simulink model "gm_transmitter"  (R2020b)
settings: Solver=FixedStepDiscrete  StartTime=0.0  StopTime=100000  RelTol=1e-3
undefined symbols (not defined in the file or in its folder): message
libraries: hdlmdlgenlib x98, dspsigops x53, hdlsllib x22, simulink x11, dspmlti4 x2, whdlio x1
(part 1 of 3)
settings Model: Creator=wardo  LastModifiedBy=EFlores
settings DataIOCC: LimitDataPoints=on  SaveOutput=off  SaveTime=off
settings OptimizationCC: BlockReduction=off  ConditionallyExecuteInputs=off  DefaultParameterBehavior=Inlined  LifeSpan=inf
settings DebuggingCC: AlgebraicLoopMsg=error  InheritedTsInSrcMsg=none  SingleTaskRateTransMsg=error  AllowSymbolicDim=off  StrictBusMsg=ErrorOnBusTreatedAsVector  SFUnexpectedBacktrackingDiag=warning  SFNoUnconditionalDefaultTransitionDiag=warning  SFExecutionAtInitializationDiag=none  ArithmeticOperatorsInVariantConditions=warning
settings HardwareCC: ProdBitPerPointer=32  ProdBitPerSizeT=32  ProdBitPerPtrDiffT=32  ProdLargestAtomicFloat=None  ProdIntDivRoundTo=Undefined  ProdEndianess=Unspecified  ProdWordSize=32  ProdHWDeviceType=ASIC/FPGA->ASIC/FPGA  ProdEqTarget=off
settings SFSimCC: SimUseLocalCustomCode=off  CustomCodeUndefinedFunction=UseInterfaceOnly
settings RTWCC: RTWUseLocalCustomCode=off
settings CodeAppCC: StateflowObjectComments=on
settings GRTTargetCC: TargetLangStandard=C89/C90 (ANSI)
settings ConfigComp: CovScope=ReferencedModels  CovMetricSettings=dw  CovSaveCumulativeToWorkspaceVar=on  CovSaveSingleToWorkspaceVar=on  CovExternalEMLEnable=off  CovSFcnEnable=off

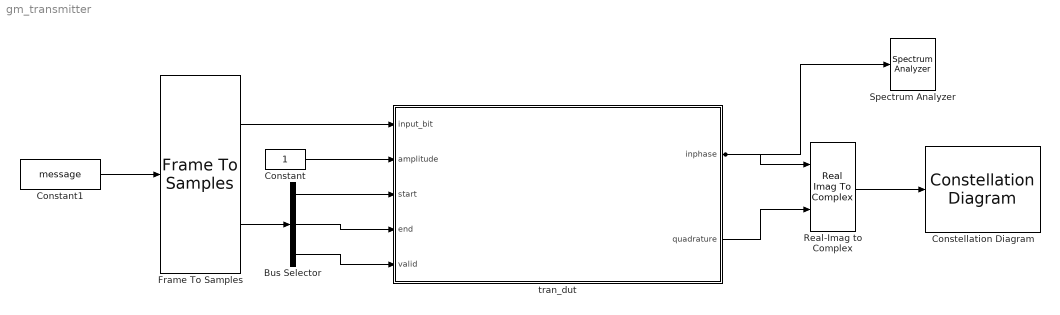
== system gm_transmitter ==
  Bus Selector : BusSelector  OutputSignals=start,end,valid
  Constant : Constant  OutDataTypeStr=uint8  SampleTime=-1
  Constant1 : Constant  Value=message  OutDataTypeStr=fixdt(0,1,0)  SampleTime=100000
  Constellation Diagram : ConstellationDiagram
  Frame To Samples : whdlio/Frame To Samples  InterSampleIdleCycles=0  InterFrameIdleCycles=0  OutputSize=1  InterleaveSamples=off
      settings: SourceProductBaseCode=LH
  Real-Imag to Complex : RealImagToComplex
  Spectrum Analyzer : SpectrumAnalyzer
  tran_dut : Subsystem
  wires:
  Bus Selector/3 -> tran_dut/5(valid)
  Bus Selector/2 -> tran_dut/4(end)
  Bus Selector/1 -> tran_dut/3(start)
  Frame To Samples/2 -> Bus Selector/1
  tran_dut/2(quadrature) -> Real-Imag to Complex/2
  tran_dut/1(inphase) -> Spectrum Analyzer/1, Real-Imag to Complex/1
  Real-Imag to Complex/1 -> Constellation Diagram/1
  Constant1/1 -> Frame To Samples/1
  Constant/1 -> tran_dut/2(amplitude)
  Frame To Samples/1 -> tran_dut/1(input_bit)

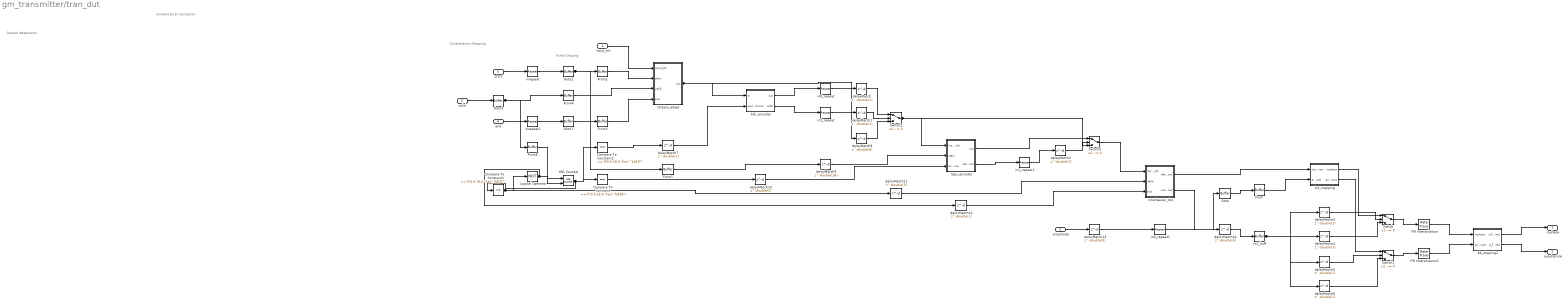
== system gm_transmitter/tran_dut ==
  note: Stream Adaptation
  note: Forward Error Correction
  note: Constellation Mapping
  note: Pulse Shaping
  input_bit : Inport  OutDataTypeStr=fixdt(0, 1, 0)  PortDimensions=1  SampleTime=2.06577425218972
  amplitude : Inport  Port=2  OutDataTypeStr=uint8  PortDimensions=1  SampleTime=2.06577425218972
  start : Inport  Port=3  OutDataTypeStr=boolean  PortDimensions=1  SampleTime=2.06577425218972
  end : Inport  Port=4  OutDataTypeStr=boolean  PortDimensions=1  SampleTime=2.06577425218972
  valid : Inport  Port=5  OutDataTypeStr=boolean  PortDimensions=1  SampleTime=2.06577425218972
  Compare To Constant : simulink/Logic and Bit Operations/Compare To Constant  relop===  const="fi(0,0,16,0,\"hex\",\"bdd8\")"  OutDataTypeStr=boolean
  Compare To Constant1 : simulink/Logic and Bit Operations/Compare To Constant  relop=<=  const="fi(0,0,16,0,\"hex\",\"fd20\")"  OutDataTypeStr=boolean
  Compare To Constant2 : simulink/Logic and Bit Operations/Compare To Constant  relop===  const="fi(0,0,16,0,\"hex\",\"bd18\")"  OutDataTypeStr=boolean
  FIR Interpolation : RateTransition  OutPortSampleTimeOpt=Multiple of input port sample time  OutPortSampleTimeMultiple=8
  FIR Interpolation1 : RateTransition  OutPortSampleTimeOpt=Multiple of input port sample time  OutPortSampleTimeMultiple=8
  From{,1..4,8} (6 alike) : hdlmdlgenlib/Buffer
      settings: SourceProductBaseCode=SL
  Goto{,1..3} (4 alike) : hdlmdlgenlib/Buffer
      settings: SourceProductBaseCode=SL
  HDL Counter : hdlsllib/Sources/HDL Counter  CountType=Count limited  CountInit=double(0)  CountStep=double(1)  CountMax=double(64800)  CountFromType=Initial value  CountFrom=double(0)  CountResetPort=on  CountLoadPort=off  CountEnbPort=on  CountDirPort=off  CountDataType=Unsigned  CountWordLen=16  CountFracLen=0  CountSampTime=2.06577425218972
  Logical Operator : Logic  Operator=NOT  Inputs=1  AllPortsSameDT=off  OutDataTypeStr=boolean  SampleTime=2.06577425218972
  Switch : Switch  Criteria=u2 ~= 0  Threshold=double(0)  OutDataTypeStr=fixdt(1, 25, 15)  SampleTime=0.258221781523715
  Switch1 : Switch  Criteria=u2 ~= 0  Threshold=double(0)  OutDataTypeStr=fixdt(1, 25, 15)  SampleTime=0.258221781523715
  Switch2 : Switch  Criteria=u2 ~= 0  Threshold=double(0)  OutDataTypeStr=boolean  SampleTime=0.258221781523715
  Switch3 : Switch  Criteria=u2 ~= 0  Threshold=double(0)  OutDataTypeStr=boolean  SampleTime=0.258221781523715
  bb_shaping1 : Subsystem
  bch_encoder : Subsystem
  bit_mapping : Subsystem
  delayMatch{,1..6} (7 alike) : Delay  DelayLength=double(1)  InitialCondition=0  SampleTime=0.258221781523715
  delayMatch10 : Delay  DelayLength=double(2)  InitialCondition=0  SampleTime=2.06577425218972
  delayMatch11 : Delay  DelayLength=double(2)  InitialCondition=0  SampleTime=2.06577425218972
  delayMatch12 : Delay  DelayLength=double(2)  InitialCondition=0  SampleTime=2.06577425218972
  delayMatch13 : Delay  DelayLength=double(3)  InitialCondition=0  SampleTime=2.06577425218972
  delayMatch14 : Delay  DelayLength=double(8)  InitialCondition=0  SampleTime=0.258221781523715
  delayMatch7 : Delay  DelayLength=double(1)  InitialCondition=0  SampleTime=2.06577425218972
  delayMatch8 : Delay  DelayLength=double(8)  InitialCondition=0  SampleTime=0.258221781523715
  delayMatch9 : Delay  DelayLength=double(16)  InitialCondition=0  SampleTime=0.258221781523715
  in0_repeat : dspsigops/Repeat  N=double(8)  RateOptions=Allow multirate processing  ic=0  mode=Unused parameter value
  in0_repeat1 : dspsigops/Repeat  N=double(8)  RateOptions=Allow multirate processing  ic=0  mode=Unused parameter value
  in1_repeat : dspsigops/Repeat  N=double(8)  RateOptions=Allow multirate processing  ic=0  mode=Unused parameter value
  in1_repeat1 : dspsigops/Repeat  N=double(8)  RateOptions=Allow multirate processing  ic=0  mode=Unused parameter value
  in2_buff : hdlmdlgenlib/Buffer
      settings: SourceProductBaseCode=SL
  inrepeat : dspsigops/Repeat  N=double(8)  RateOptions=Allow multirate processing  ic=0  mode=Unused parameter value
  inrepeat1 : dspsigops/Repeat  N=double(8)  RateOptions=Allow multirate processing  ic=0  mode=Unused parameter value
  interleaver_dut : Subsystem
  ldpc_encoder : Subsystem
  stream_adapt : Subsystem
  inphase : Outport  VectorParamsAs1DForOutWhenUnconnected=off
  quadrature : Outport  Port=2  VectorParamsAs1DForOutWhenUnconnected=off
  wires:
  input_bit/1 -> stream_adapt/1(input_bit)
  delayMatch13/1 -> in0_repeat1/1
  start/1 -> inrepeat/1
  end/1 -> inrepeat1/1
  valid/1 -> Goto3/1
  HDL Counter/1 -> Compare To Constant1/1, Compare To Constant2/1, Compare To Constant/1
  bb_shaping1/1(i_filtered) -> inphase/1
  bb_shaping1/2(q_filtered) -> quadrature/1
  bch_encoder/1(out) -> in0_repeat/1
  bch_encoder/2(valid) -> in1_repeat/1
  interleaver_dut/1(data_out) -> bit_mapping/1(input_sequence)
  delayMatch14/1 -> in2_buff/1
  ldpc_encoder/1(out) -> Switch3/1
  ldpc_encoder/2(valid_out) -> in1_repeat1/1
  delayMatch8/1 -> Switch2/3
  From2/1 -> stream_adapt/2(start)
  delayMatch9/1 -> ldpc_encoder/2(start)
  From4/1 -> stream_adapt/3(valid)
  From8/1 -> HDL Counter/2
  From3/1 -> stream_adapt/4(end)
  delayMatch11/1 -> interleaver_dut/2(valid)
  delayMatch12/1 -> interleaver_dut/3(end)
  delayMatch7/1 -> bch_encoder/2(end_of_frame)
  Switch2/1 -> ldpc_encoder/1(input_bit), Switch3/3
  delayMatch10/1 -> ldpc_encoder/3(end_of_frame)
  Switch3/1 -> interleaver_dut/1(input_bit)
  FIR Interpolation/1 -> bb_shaping1/1(inphase)
  FIR Interpolation1/1 -> bb_shaping1/2(quadrature)
  Compare To Constant2/1 -> delayMatch7/1
  stream_adapt/1(out) -> delayMatch8/1, bch_encoder/1(in)
  From1/1 -> delayMatch9/1
  Compare To Constant/1 -> delayMatch10/1
  Compare To Constant1/1 -> delayMatch11/1, Logical Operator/1
  Logical Operator/1 -> delayMatch12/1, HDL Counter/1
  amplitude/1 -> delayMatch13/1
  interleaver_dut/2(valid_out) -> delayMatch14/1
  inrepeat/1 -> Goto2/1
  Goto2/1 -> From2/1, From1/1
  Goto3/1 -> From8/1, From4/1
  inrepeat1/1 -> Goto1/1
  Goto1/1 -> From3/1
  in0_repeat/1 -> delayMatch/1
  in1_repeat/1 -> delayMatch1/1
  delayMatch/1 -> Switch2/1
  delayMatch1/1 -> Switch2/2
  in1_repeat1/1 -> delayMatch2/1
  delayMatch2/1 -> Switch3/2
  Switch/1 -> FIR Interpolation/1
  Switch1/1 -> FIR Interpolation1/1
  in0_repeat1/1 -> Goto/1
  Goto/1 -> From/1
  From/1 -> bit_mapping/2(amplitude)
  bit_mapping/1(inphase) -> Switch/1
  bit_mapping/2(quadrature) -> Switch1/1
  delayMatch3/1 -> Switch/2
  delayMatch4/1 -> Switch/3
  delayMatch5/1 -> Switch1/2
  delayMatch6/1 -> Switch1/3
  in2_buff/1 -> delayMatch6/1, delayMatch5/1, delayMatch4/1, delayMatch3/1

== system gm_transmitter/tran_dut/bb_shaping1 ==
  inphase : Inport  OutDataTypeStr=fixdt(1, 25, 15)  PortDimensions=1  SampleTime=2.06577425218972
  quadrature : Inport  Port=2  OutDataTypeStr=fixdt(1, 25, 15)  PortDimensions=1  SampleTime=2.06577425218972
  FIR Interpolation : dspmlti4/FIR Interpolation  FilterSource=Dialog parameters  PrivateCoeffs=0  h=[-0.00599670410156250,-0.00514221191406250,-0.00289916992187500,0.000442504882812500,0.00431823730468750,0.00794982910156250,0.0104980468750000,0.0112304687500000,0.00967407226562500,0.00578308105468750,0,-0.00680541992187500,-0.0134124755859375,-0.0184326171875000,-0.0205841064453125,-0.0189819335937500,-0.0133361816406250,-0.00410461425781250,0.00752258300781250,0.0196380615234375,0.0300140380859375,0.0363464355468750,0.0367584228515625,0.0301208496093750,0.0164794921875000,-0.00291442871093750,-0.0254821777343750,-0.0476837158203125,-0.0653228759765625,-0.0742187500000000,-0.0707244873046875,-0.0524291992187500,-0.0185852050781250,0.0296783447265625,0.0892028808593750,0.155227661132813,0.221755981445313,0.282333374023438,0.330810546875000,0.362121582031250,0.372940063476563,0.362121582031250,0.330810546875000,0.282333374023438,0.221755981445313,0.155227661132813,0.0892028808593750,0.0296783447265625,-0.0185852050781250,-0.0524291992187500,-0.0707244873046875,-0.0742187500000000,-0.0653228759765625,-0.0476837158203125,-0.0254821777343750,-0.00291442871093750,0.0164794921875000,0.0301208496093750,0.0367584228515625,0.0363464355468750,0.0300140380859375,0.0196380615234375,0.00752258300781250,-0.00410461425781250,-0.0133361816406250,-0.0189819335937500,-0.0205841064453125,-0.0184326171875000,-0.0134124755859375,-0.00680541992187500,0,0.00578308105468750,0.00967407226562500,0.0112304687500000,0.0104980468750000,0.00794982910156250,0.00431823730468750,0.000442504882812500,-0.00289916992187500,-0.00514221191406250,-0.00599670410156250]  L=8  FilterObject=FINTERP  framing=Allow multirate processing  outputBufInitCond=0  roundingMode=Floor  overflowMode=off  firstCoeffMode=Specify word length  firstCoeffWordLength=16  firstCoeffFracLength=15  firstCoeffDataTypeStr=fixdt(1,16)  firstCoeffMin=[]  firstCoeffMax=[]  firstCoeffLastDataTypeStr=fixdt(1,16)  outputDataTypeStr=Inherit: Same as accumulator  outputMin=[]  outputMax=[]  outputLastDataTypeStr=Inherit: Same as accumulator
      settings: SourceProductName=DSP System Toolbox
  FIR Interpolation1 : dspmlti4/FIR Interpolation  FilterSource=Dialog parameters  PrivateCoeffs=0  h=[-0.00599670410156250,-0.00514221191406250,-0.00289916992187500,0.000442504882812500,0.00431823730468750,0.00794982910156250,0.0104980468750000,0.0112304687500000,0.00967407226562500,0.00578308105468750,0,-0.00680541992187500,-0.0134124755859375,-0.0184326171875000,-0.0205841064453125,-0.0189819335937500,-0.0133361816406250,-0.00410461425781250,0.00752258300781250,0.0196380615234375,0.0300140380859375,0.0363464355468750,0.0367584228515625,0.0301208496093750,0.0164794921875000,-0.00291442871093750,-0.0254821777343750,-0.0476837158203125,-0.0653228759765625,-0.0742187500000000,-0.0707244873046875,-0.0524291992187500,-0.0185852050781250,0.0296783447265625,0.0892028808593750,0.155227661132813,0.221755981445313,0.282333374023438,0.330810546875000,0.362121582031250,0.372940063476563,0.362121582031250,0.330810546875000,0.282333374023438,0.221755981445313,0.155227661132813,0.0892028808593750,0.0296783447265625,-0.0185852050781250,-0.0524291992187500,-0.0707244873046875,-0.0742187500000000,-0.0653228759765625,-0.0476837158203125,-0.0254821777343750,-0.00291442871093750,0.0164794921875000,0.0301208496093750,0.0367584228515625,0.0363464355468750,0.0300140380859375,0.0196380615234375,0.00752258300781250,-0.00410461425781250,-0.0133361816406250,-0.0189819335937500,-0.0205841064453125,-0.0184326171875000,-0.0134124755859375,-0.00680541992187500,0,0.00578308105468750,0.00967407226562500,0.0112304687500000,0.0104980468750000,0.00794982910156250,0.00431823730468750,0.000442504882812500,-0.00289916992187500,-0.00514221191406250,-0.00599670410156250]  L=8  FilterObject=FINTERP  framing=Allow multirate processing  outputBufInitCond=0  roundingMode=Floor  overflowMode=off  firstCoeffMode=Specify word length  firstCoeffWordLength=16  firstCoeffFracLength=15  firstCoeffDataTypeStr=fixdt(1,16)  firstCoeffMin=[]  firstCoeffMax=[]  firstCoeffLastDataTypeStr=fixdt(1,16)  outputDataTypeStr=Inherit: Same as accumulator  outputMin=[]  outputMax=[]  outputLastDataTypeStr=Inherit: Same as accumulator
      settings: SourceProductName=DSP System Toolbox
  i_filtered : Outport  VectorParamsAs1DForOutWhenUnconnected=off
  q_filtered : Outport  Port=2  VectorParamsAs1DForOutWhenUnconnected=off
  wires:
  FIR Interpolation/1 -> i_filtered/1
  FIR Interpolation1/1 -> q_filtered/1
  inphase/1 -> FIR Interpolation/1
  quadrature/1 -> FIR Interpolation1/1

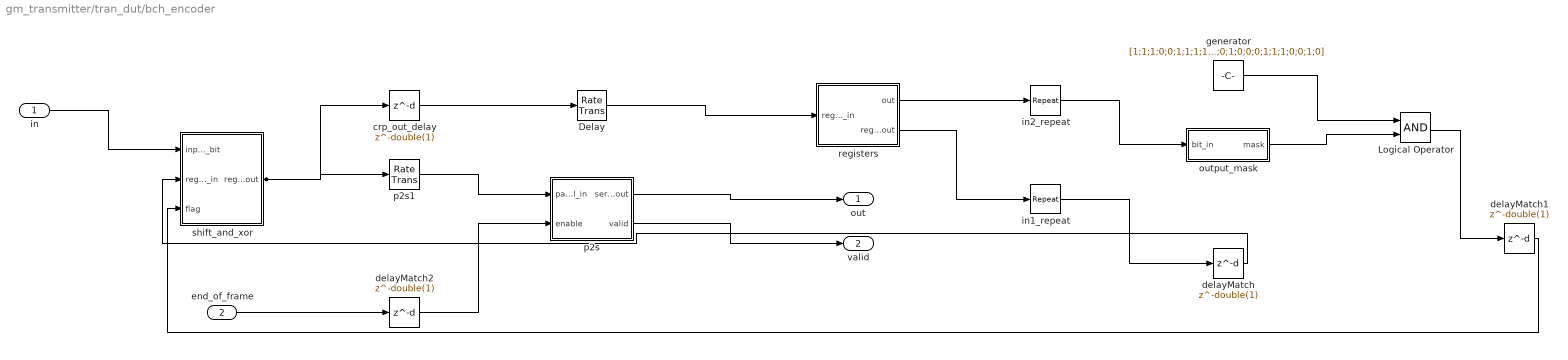
== system gm_transmitter/tran_dut/bch_encoder ==
  in : Inport  OutDataTypeStr=boolean  PortDimensions=1  SampleTime=0.258221781523715
  end_of_frame : Inport  Port=2  OutDataTypeStr=boolean  PortDimensions=1  SampleTime=2.06577425218972
  Delay : RateTransition  OutPortSampleTimeOpt=Multiple of input port sample time  OutPortSampleTimeMultiple=8
  Logical Operator : Logic  AllPortsSameDT=off  OutDataTypeStr=fixdt(0, 1, 0)  SampleTime=0.258221781523715
  crp_out_delay : Delay  DelayLength=double(1)  InitialCondition=0  SampleTime=0.258221781523715
  delayMatch : Delay  DelayLength=double(1)  InitialCondition=0  SampleTime=0.258221781523715
  delayMatch1 : Delay  DelayLength=double(1)  InitialCondition=0  SampleTime=0.258221781523715
  delayMatch2 : Delay  DelayLength=double(1)  InitialCondition=0  SampleTime=2.06577425218972
  generator : Constant  Value=[1;1;1;0;0;1;1;1;1;0;1;0;1;0;1;0;0;1;0;0;0;0;0;0;0;1;1;0;0;1;1;0;1;1;1;0;1;1;1;1;1;0;1;0;0;0;0;1;1;1;1;0;0;0;1;0;1;1;0;0;0;0;0;0;1;0;0;1;0;0;0;1;0;0;0;1;0;0;0;0;1;0;1;0;1;1;0;0;0;0;1;1;1;0;1;1;0;0;0;1;1;0;1;1;0;0;1;1;0;1;0;0;1;1;1;1;0;0;1;1;0;0;0;0;1;0;1;0;0;0;1;1;1;0;0;0;1;0;0;0;1;0;1;0;0;0;1;1;1;0;1;0;0;0;1;0;0;0;0;1;1;1;0;0;0;0;0;1;0;1;1;1;0;0;0;0;0;1;1;0;0;1;0;0;0;1;1;1;0;0;1;0]  OutDataTypeStr=fixdt(0, 1, 0)  SampleTime=0.258221781523715
  in1_repeat : dspsigops/Repeat  N=double(8)  RateOptions=Allow multirate processing  ic=0  mode=Unused parameter value
  in2_repeat : dspsigops/Repeat  N=double(8)  RateOptions=Allow multirate processing  ic=0  mode=Unused parameter value
  output_mask : Subsystem
  p2s : Subsystem
  p2s1 : RateTransition  OutPortSampleTimeOpt=Multiple of input port sample time  OutPortSampleTimeMultiple=8
  registers : Subsystem
  shift_and_xor : Subsystem
  out : Outport  VectorParamsAs1DForOutWhenUnconnected=off
  valid : Outport  Port=2  VectorParamsAs1DForOutWhenUnconnected=off
  wires:
  p2s/1(serial_out) -> out/1
  p2s/2(valid) -> valid/1
  delayMatch2/1 -> p2s/2(enable)
  in/1 -> shift_and_xor/1(input_bit)
  end_of_frame/1 -> delayMatch2/1
  registers/1(out) -> in2_repeat/1
  registers/2(registers_out) -> in1_repeat/1
  Delay/1 -> registers/1(registers_in)
  p2s1/1 -> p2s/1(parallel_in)
  crp_out_delay/1 -> Delay/1
  shift_and_xor/1(registers_out) -> p2s1/1, crp_out_delay/1
  in1_repeat/1 -> delayMatch/1
  in2_repeat/1 -> output_mask/1(bit_in)
  generator/1 -> Logical Operator/1
  output_mask/1(mask) -> Logical Operator/2
  delayMatch1/1 -> shift_and_xor/3(flag)
  delayMatch/1 -> shift_and_xor/2(registers_in)
  Logical Operator/1 -> delayMatch1/1

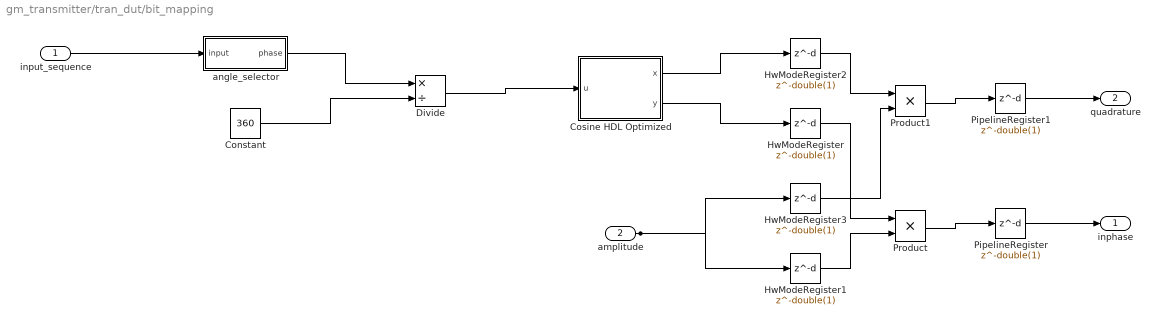
== system gm_transmitter/tran_dut/bit_mapping ==
  input_sequence : Inport  OutDataTypeStr=fixdt(0, 3, 0)  PortDimensions=1  SampleTime=0.258221781523715
  amplitude : Inport  Port=2  OutDataTypeStr=uint8  PortDimensions=1  SampleTime=0.258221781523715
  Constant : Constant  Value=360  OutDataTypeStr=fixdt(0, 9, 0)  SampleTime=0.258221781523715
  Cosine HDL Optimized : Subsystem  mask(Sine and Cosine HDL optimized block){OutputFormula=sin(2*pi*u) and cos(2*pi*u), NumDataPoints=double(32), TableDataTypeStr=fixdt(1,16,15), SimulateLUTROMDelay=off}
      mask prompts: OutputFormula "Simulink:masks:OutputFormula_MP"; NumDataPoints "HDLShared:hdlshared:CosineHDL_Npts"; TableDataTypeStr "Simulink:blkprm_prompts:TABLE_UNIFIEDDATATYPE"; SimulateLUTROMDelay "HDLShared:hdlshared:CosineHDL_Map2RAM"
      mask help: Sine and Cosine HDL optimized block using quarter wave symmetry, and HDL friendly settings.
      mask Help: helpview([docroot '/hdlcoder/helptargets.map'],'SineAndCosineHDL_Optimized');
      mask TypeOptions OutputFormula: sin(2*pi*u) | cos(2*pi*u) | exp(j*2*pi*u) | sin(2*pi*u) and cos(2*pi*u)
      mask Display:
      | port_label('input',1,'u')
      | port_label('output',1,'sin(2*pi*u)')
      | port_label('output',2,'cos(2*pi*u)')
      | xpos = 0.35;
      | yoffset = 0.5;
      | if ( SimulateLUTROMDelay )
      |   text(xpos,yoffset,'HDL (Z^{-1})','texmode','on')
      | else
      |    text(xpos,yoffset,'HDL')
      | end
  Divide : Product  Inputs=*/  OutDataTypeStr=fixdt(1, 16, 14)  RndMeth=Zero  SaturateOnIntegerOverflow=on  SampleTime=0.258221781523715
  HwModeRegister{,1..3} (4 alike) : Delay  DelayLength=double(1)  InitialCondition=0  SampleTime=0.258221781523715
  PipelineRegister : Delay  DelayLength=double(1)  InitialCondition=0  SampleTime=0.258221781523715
  PipelineRegister1 : Delay  DelayLength=double(1)  InitialCondition=0  SampleTime=0.258221781523715
  Product : Product  Inputs=**  OutDataTypeStr=fixdt(1, 25, 15)  SampleTime=0.258221781523715
  Product1 : Product  Inputs=**  OutDataTypeStr=fixdt(1, 25, 15)  SampleTime=0.258221781523715
  angle_selector : Subsystem
  inphase : Outport  VectorParamsAs1DForOutWhenUnconnected=off
  quadrature : Outport  Port=2  VectorParamsAs1DForOutWhenUnconnected=off
  wires:
  Constant/1 -> Divide/2
  Cosine HDL Optimized/1(x) -> HwModeRegister2/1
  Cosine HDL Optimized/2(y) -> HwModeRegister/1
  Divide/1 -> Cosine HDL Optimized/1(u)
  PipelineRegister/1 -> inphase/1
  PipelineRegister1/1 -> quadrature/1
  angle_selector/1(phase) -> Divide/1
  input_sequence/1 -> angle_selector/1(input)
  amplitude/1 -> HwModeRegister1/1, HwModeRegister3/1
  Product/1 -> PipelineRegister/1
  HwModeRegister/1 -> Product/1
  HwModeRegister1/1 -> Product/2
  Product1/1 -> PipelineRegister1/1
  HwModeRegister2/1 -> Product1/1
  HwModeRegister3/1 -> Product1/2

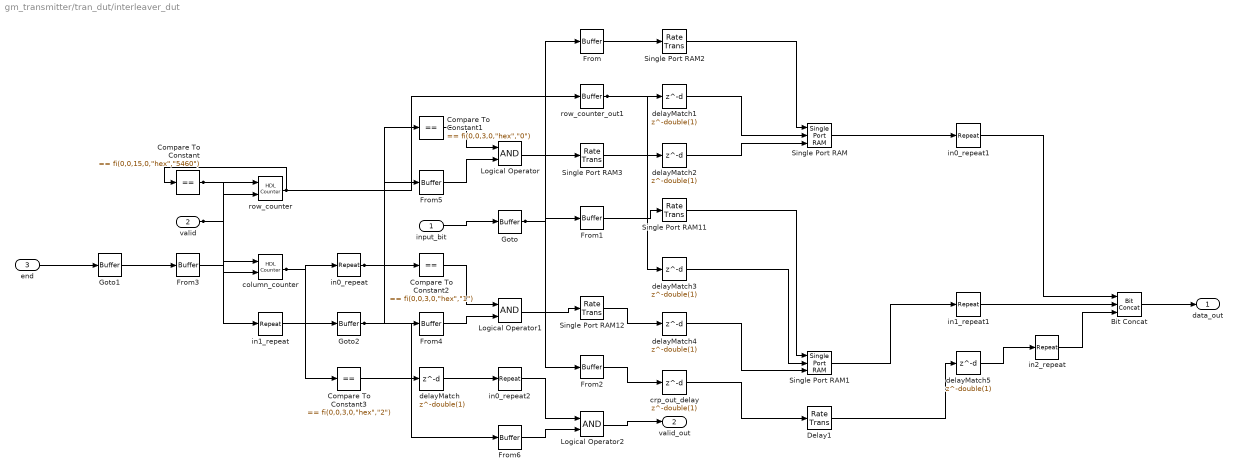
== system gm_transmitter/tran_dut/interleaver_dut ==
  input_bit : Inport  OutDataTypeStr=boolean  PortDimensions=1  SampleTime=0.258221781523715
  valid : Inport  Port=2  OutDataTypeStr=boolean  PortDimensions=1  SampleTime=2.06577425218972
  end : Inport  Port=3  OutDataTypeStr=boolean  PortDimensions=1  SampleTime=2.06577425218972
  Bit Concat : hdlsllib/Logic and Bit Operations/Bit Concat  numInputs=3
  Compare To Constant : simulink/Logic and Bit Operations/Compare To Constant  relop===  const="fi(0,0,15,0,\"hex\",\"5460\")"  OutDataTypeStr=boolean
  Compare To Constant1 : simulink/Logic and Bit Operations/Compare To Constant  relop===  const="fi(0,0,3,0,\"hex\",\"0\")"  OutDataTypeStr=boolean
  Compare To Constant2 : simulink/Logic and Bit Operations/Compare To Constant  relop===  const="fi(0,0,3,0,\"hex\",\"1\")"  OutDataTypeStr=boolean
  Compare To Constant3 : simulink/Logic and Bit Operations/Compare To Constant  relop===  const="fi(0,0,3,0,\"hex\",\"2\")"  OutDataTypeStr=boolean
  Delay1 : RateTransition  OutPortSampleTimeOpt=Multiple of input port sample time  OutPortSampleTimeMultiple=8
  From{,1..6} (7 alike) : hdlmdlgenlib/Buffer
      settings: SourceProductBaseCode=SL
  Goto : hdlmdlgenlib/Buffer
      settings: SourceProductBaseCode=SL
  Goto1 : hdlmdlgenlib/Buffer
      settings: SourceProductBaseCode=SL
  Goto2 : hdlmdlgenlib/Buffer
      settings: SourceProductBaseCode=SL
  Logical Operator : Logic  AllPortsSameDT=off  OutDataTypeStr=boolean  SampleTime=0.258221781523715
  Logical Operator1 : Logic  AllPortsSameDT=off  OutDataTypeStr=boolean  SampleTime=0.258221781523715
  Logical Operator2 : Logic  AllPortsSameDT=off  OutDataTypeStr=boolean  SampleTime=0.258221781523715
  Single Port RAM : hdlsllib/HDL RAMs/Single Port RAM  ram_size=15  dout_type=New data
      settings: SourceProductBaseCode=SL
  Single Port RAM1 : hdlsllib/HDL RAMs/Single Port RAM  ram_size=15  dout_type=New data
      settings: SourceProductBaseCode=SL
  Single Port RAM{2..3,11..12} (4 alike) : RateTransition  OutPortSampleTimeOpt=Multiple of input port sample time  OutPortSampleTimeMultiple=8
  column_counter : hdlsllib/Sources/HDL Counter  CountType=Count limited  CountInit=double(0)  CountStep=double(1)  CountMax=double(2)  CountFromType=Initial value  CountFrom=double(0)  CountResetPort=on  CountLoadPort=off  CountEnbPort=on  CountDirPort=off  CountDataType=Unsigned  CountWordLen=3  CountFracLen=0  CountSampTime=2.06577425218972
  crp_out_delay : Delay  DelayLength=double(1)  InitialCondition=0  SampleTime=0.258221781523715
  delayMatch{,1..5} (6 alike) : Delay  DelayLength=double(1)  InitialCondition=0  SampleTime=2.06577425218972
  in0_repeat : dspsigops/Repeat  N=double(8)  RateOptions=Allow multirate processing  ic=0  mode=Unused parameter value
  in0_repeat1 : dspsigops/Repeat  N=double(8)  RateOptions=Allow multirate processing  ic=0  mode=Unused parameter value
  in0_repeat2 : dspsigops/Repeat  N=double(8)  RateOptions=Allow multirate processing  ic=0  mode=Unused parameter value
  in1_repeat : dspsigops/Repeat  N=double(8)  RateOptions=Allow multirate processing  ic=0  mode=Unused parameter value
  in1_repeat1 : dspsigops/Repeat  N=double(8)  RateOptions=Allow multirate processing  ic=0  mode=Unused parameter value
  in2_repeat : dspsigops/Repeat  N=double(8)  RateOptions=Allow multirate processing  ic=0  mode=Unused parameter value
  row_counter : hdlsllib/Sources/HDL Counter  CountType=Count limited  CountInit=double(1)  CountStep=double(1)  CountMax=double(21600)  CountFromType=Initial value  CountFrom=double(1)  CountResetPort=on  CountLoadPort=off  CountEnbPort=on  CountDirPort=off  CountDataType=Unsigned  CountWordLen=15  CountFracLen=0  CountSampTime=2.06577425218972
  row_counter_out1 : hdlmdlgenlib/Buffer
      settings: SourceProductBaseCode=SL
  data_out : Outport  VectorParamsAs1DForOutWhenUnconnected=off
  valid_out : Outport  Port=2  VectorParamsAs1DForOutWhenUnconnected=off
  wires:
  delayMatch/1 -> in0_repeat2/1
  delayMatch5/1 -> in2_repeat/1
  Single Port RAM/1 -> in0_repeat1/1
  Single Port RAM1/1 -> in1_repeat1/1
  column_counter/1 -> in0_repeat/1, Compare To Constant3/1
  delayMatch1/1 -> Single Port RAM/2
  From3/1 -> column_counter/1
  delayMatch2/1 -> Single Port RAM/3
  delayMatch4/1 -> Single Port RAM1/3
  From6/1 -> Logical Operator2/2
  Bit Concat/1 -> data_out/1
  Logical Operator2/1 -> valid_out/1
  Single Port RAM2/1 -> Single Port RAM/1
  Single Port RAM11/1 -> Single Port RAM1/1
  input_bit/1 -> Goto/1
  valid/1 -> row_counter/2, in1_repeat/1
  end/1 -> Goto1/1
  delayMatch3/1 -> Single Port RAM1/2
  Single Port RAM3/1 -> delayMatch2/1
  row_counter_out1/1 -> delayMatch3/1, delayMatch1/1
  Single Port RAM12/1 -> delayMatch4/1
  Delay1/1 -> delayMatch5/1
  Compare To Constant/1 -> row_counter/1, column_counter/2
  row_counter/1 -> row_counter_out1/1, Compare To Constant/1
  From/1 -> Single Port RAM2/1
  From1/1 -> Single Port RAM11/1
  crp_out_delay/1 -> Delay1/1
  Goto/1 -> From2/1, From1/1, From/1
  From2/1 -> crp_out_delay/1
  Goto1/1 -> From3/1
  Logical Operator/1 -> Single Port RAM3/1
  Logical Operator1/1 -> Single Port RAM12/1
  in0_repeat/1 -> Compare To Constant2/1, Compare To Constant1/1
  in1_repeat/1 -> Goto2/1
  Compare To Constant1/1 -> Logical Operator/1
  Goto2/1 -> From6/1, From5/1, From4/1
  From5/1 -> Logical Operator/2
  Compare To Constant2/1 -> Logical Operator1/1
  From4/1 -> Logical Operator1/2
  in0_repeat1/1 -> Bit Concat/1
  in1_repeat1/1 -> Bit Concat/2
  in2_repeat/1 -> Bit Concat/3
  Compare To Constant3/1 -> delayMatch/1
  in0_repeat2/1 -> Logical Operator2/1

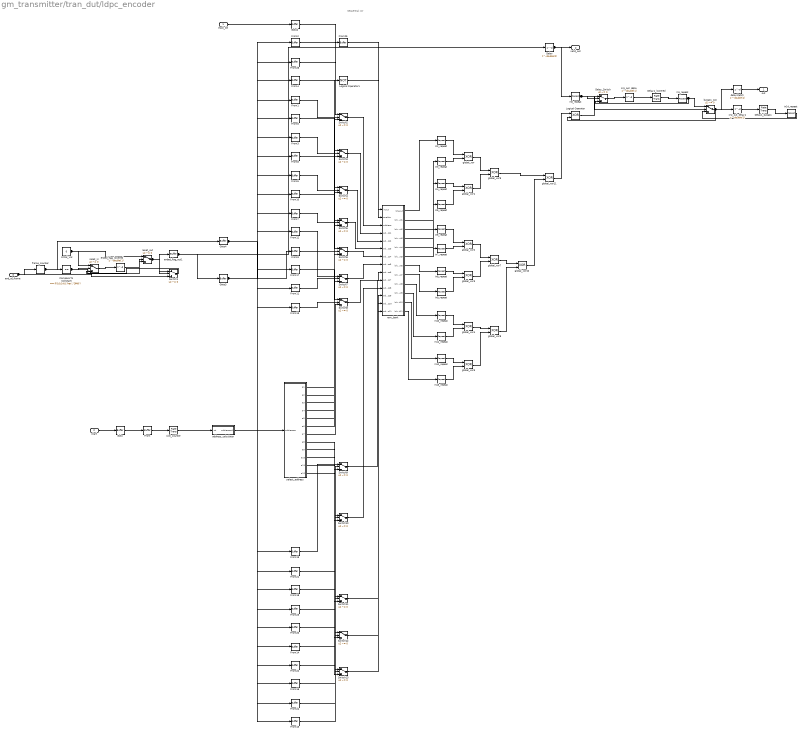
== system gm_transmitter/tran_dut/ldpc_encoder ==
  note: Sequential xor
  input_bit : Inport  OutDataTypeStr=boolean  PortDimensions=1  SampleTime=0.258221781523715
  start : Inport  Port=2  OutDataTypeStr=boolean  PortDimensions=1  SampleTime=0.258221781523715
  end_of_frame : Inport  Port=3  OutDataTypeStr=boolean  PortDimensions=1  SampleTime=2.06577425218972
  Compare To Constant : simulink/Logic and Bit Operations/Compare To Constant  relop===  const="fi(0,0,14,0,\"hex\",\"3f48\")"  OutDataTypeStr=boolean
  Delay : Delay  DelayLength=double(2)  InitialCondition=0  SampleTime=2.06577425218972
  Delay1_bypass : RateTransition  OutPortSampleTimeOpt=Multiple of input port sample time  OutPortSampleTimeMultiple=8
  Delay1_lowered : RateTransition  OutPortSampleTimeOpt=Multiple of input port sample time  OutPortSampleTimeMultiple=8
  Delay_Switch : Switch  Criteria=u2 ~= 0  Threshold=double(0)  OutDataTypeStr=fixdt(0, 1, 0)  SampleTime=0.258221781523715
  From{,1..26} (27 alike) : hdlmdlgenlib/Buffer
      settings: SourceProductBaseCode=SL
  Goto{,2..4} (4 alike) : hdlmdlgenlib/Buffer
      settings: SourceProductBaseCode=SL
  Initial_Val : Constant  Value=0  OutDataTypeStr=boolean  SampleTime=2.06577425218972
  Logical Operator : Logic  Operator=XOR  AllPortsSameDT=off  OutDataTypeStr=fixdt(0, 1, 0)  SampleTime=0.258221781523715
  Logical Operator1 : Logic  Operator=NOT  Inputs=1  AllPortsSameDT=off  OutDataTypeStr=boolean  SampleTime=2.06577425218972
  Switch1 : Switch  Criteria=u2 ~= 0  Threshold=double(0)  OutDataTypeStr=boolean  SampleTime=2.06577425218972
  Switch{2..13} (12 alike) : Switch  Criteria=u2 ~= 0  Threshold=double(0)  OutDataTypeStr=fixdt(0, 14, 0)  SampleTime=2.06577425218972
  address_calculator : Subsystem
  bypass_out : Switch  Criteria=u2 ~= 0  Threshold=double(0)  OutDataTypeStr=fixdt(0, 1, 0)  SampleTime=0.258221781523715
  crp_out_delay : Delay  DelayLength=double(1)  InitialCondition=0  SampleTime=0.258221781523715
  crp_out_delay1 : Delay  DelayLength=double(1)  InitialCondition=0  SampleTime=0.258221781523715
  delayMatch : Delay  DelayLength=double(1)  InitialCondition=0  SampleTime=0.258221781523715
  ended_flag_lowered : Delay  DelayLength=double(1)  InitialCondition=0  SampleTime=2.06577425218972
  ended_flag_out1 : hdlmdlgenlib/Buffer
      settings: SourceProductBaseCode=SL
  frame_counter : hdlsllib/Sources/HDL Counter  CountType=Count limited  CountInit=double(0)  CountStep=double(1)  CountMax=double(16200)  CountFromType=Initial value  CountFrom=double(0)  CountResetPort=on  CountLoadPort=off  CountEnbPort=off  CountDirPort=off  CountDataType=Unsigned  CountWordLen=14  CountFracLen=0  CountSampTime=2.06577425218972
  global_xor{,1..5,7..11} (11 alike) : Logic  Operator=XOR  AllPortsSameDT=off  OutDataTypeStr=boolean  SampleTime=0.258221781523715
  in0_repeat : dspsigops/Repeat  N=double(8)  RateOptions=Allow multirate processing  ic=0  mode=Unused parameter value
  in10_repeat : dspsigops/Repeat  N=double(8)  RateOptions=Allow multirate processing  ic=0  mode=Unused parameter value
  in11_repeat : dspsigops/Repeat  N=double(8)  RateOptions=Allow multirate processing  ic=0  mode=Unused parameter value
  in12_repeat : dspsigops/Repeat  N=double(8)  RateOptions=Allow multirate processing  ic=0  mode=Unused parameter value
  in13_repeat : dspsigops/Repeat  N=double(8)  RateOptions=Allow multirate processing  ic=0  mode=Unused parameter value
  in14_repeat : dspsigops/Repeat  N=double(8)  RateOptions=Allow multirate processing  ic=0  mode=Unused parameter value
  in1_repeat : dspsigops/Repeat  N=double(8)  RateOptions=Allow multirate processing  ic=0  mode=Unused parameter value
  in2_repeat : dspsigops/Repeat  N=double(8)  RateOptions=Allow multirate processing  ic=0  mode=Unused parameter value
  in3_repeat : dspsigops/Repeat  N=double(8)  RateOptions=Allow multirate processing  ic=0  mode=Unused parameter value
  in4_repeat : dspsigops/Repeat  N=double(8)  RateOptions=Allow multirate processing  ic=0  mode=Unused parameter value
  in5_repeat : dspsigops/Repeat  N=double(8)  RateOptions=Allow multirate processing  ic=0  mode=Unused parameter value
  in6_repeat : dspsigops/Repeat  N=double(8)  RateOptions=Allow multirate processing  ic=0  mode=Unused parameter value
  in7_repeat : dspsigops/Repeat  N=double(8)  RateOptions=Allow multirate processing  ic=0  mode=Unused parameter value
  in8_repeat : dspsigops/Repeat  N=double(8)  RateOptions=Allow multirate processing  ic=0  mode=Unused parameter value
  in9_repeat : dspsigops/Repeat  N=double(8)  RateOptions=Allow multirate processing  ic=0  mode=Unused parameter value
  ram_bank : Subsystem
  reset_in : Switch  Criteria=u2 ~= 0  Threshold=double(0)  OutDataTypeStr=boolean  SampleTime=2.06577425218972
  reset_out : Switch  Criteria=u2 ~= 0  Threshold=double(0)  OutDataTypeStr=boolean  SampleTime=2.06577425218972
  select_address : Subsystem
  slot_counter : RateTransition  OutPortSampleTimeOpt=Multiple of input port sample time  OutPortSampleTimeMultiple=8
  out : Outport  VectorParamsAs1DForOutWhenUnconnected=off
  valid_out : Outport  Port=2  VectorParamsAs1DForOutWhenUnconnected=off
  wires:
  Delay/1 -> valid_out/1, in0_repeat/1
  Switch10/1 -> ram_bank/11(address8)
  Switch11/1 -> ram_bank/12(address9)
  Switch12/1 -> ram_bank/13(address10)
  Switch13/1 -> ram_bank/14(address11)
  Switch2/1 -> ram_bank/3(address)
  Switch3/1 -> ram_bank/4(address1)
  Switch4/1 -> ram_bank/5(address2)
  Switch5/1 -> ram_bank/6(address3)
  Switch6/1 -> ram_bank/7(address4)
  Switch7/1 -> ram_bank/8(address5)
  Switch8/1 -> ram_bank/9(address6)
  Switch9/1 -> ram_bank/10(address7)
  address_calculator/1(addresses1) -> select_address/1(addresses)
  ended_flag_out1/1 -> Delay/1, Goto3/1
  frame_counter/1 -> Compare To Constant/1, Goto4/1
  ram_bank/1(bit_out) -> in2_repeat/1
  ram_bank/2(bit_out1) -> in3_repeat/1
  ram_bank/3(bit_out2) -> in4_repeat/1
  ram_bank/4(bit_out3) -> in5_repeat/1
  ram_bank/5(bit_out4) -> in6_repeat/1
  ram_bank/6(bit_out5) -> in7_repeat/1
  ram_bank/7(bit_out6) -> in8_repeat/1
  ram_bank/8(bit_out7) -> in9_repeat/1
  ram_bank/9(bit_out8) -> in10_repeat/1
  ram_bank/10(bit_out9) -> in11_repeat/1
  ram_bank/11(bit_out10) -> in12_repeat/1
  ram_bank/12(bit_out11) -> in13_repeat/1
  Logical Operator1/1 -> ram_bank/2(enable)
  From7/1 -> Switch5/2
  From2/1 -> Switch2/1
  From1/1 -> Switch2/2
  From4/1 -> Switch3/1
  From3/1 -> Switch3/2
  From6/1 -> Switch4/1
  From5/1 -> Switch4/2
  From12/1 -> Switch7/1
  From11/1 -> Switch7/2
  From17/1 -> Switch8/1
  From13/1 -> Switch8/2
  From19/1 -> Switch9/1
  From18/1 -> Switch9/2
  From21/1 -> Switch10/1
  From20/1 -> Switch10/2
  From23/1 -> Switch11/1
  From22/1 -> Switch11/2
  From14/1 -> Switch12/1
  From24/1 -> Switch12/2
  From16/1 -> Switch13/1
  From15/1 -> Switch13/2
  select_address/1(a1) -> Switch2/3
  select_address/2(a2) -> Switch3/3
  select_address/3(a3) -> Switch4/3
  select_address/4(a4) -> Switch5/3
  select_address/5(a5) -> Switch6/3
  select_address/6(a6) -> Switch7/3
  select_address/7(a7) -> Switch8/3
  select_address/8(a8) -> Switch9/3
  select_address/9(a9) -> Switch10/3
  select_address/10(a10) -> Switch11/3
  select_address/11(a11) -> Switch12/3
  select_address/12(a12) -> Switch13/3
  From8/1 -> Switch5/1
  Goto4/1 -> From8/1, From6/1, From4/1, From23/1, From21/1, From2/1, From19/1, From17/1, From16/1, From14/1, From12/1, From10/1
  From10/1 -> Switch6/1
  From9/1 -> Switch6/2
  From26/1 -> Logical Operator1/1
  Goto3/1 -> From9/1, From7/1, From5/1, From3/1, From26/1, From24/1, From22/1, From20/1, From18/1, From15/1, From13/1, From11/1, From1/1
  Initial_Val/1 -> reset_out/1, reset_in/1
  Compare To Constant/1 -> reset_out/2, reset_in/2
  slot_counter/1 -> address_calculator/1(rst)
  From25/1 -> ram_bank/1(input)
  input_bit/1 -> Goto2/1
  start/1 -> Goto/1
  end_of_frame/1 -> frame_counter/1, Switch1/3
  Switch1/1 -> reset_in/3
  reset_in/1 -> ended_flag_lowered/1
  ended_flag_lowered/1 -> reset_out/3
  reset_out/1 -> ended_flag_out1/1, Switch1/2, Switch1/1
  Delay1_lowered/1 -> in1_repeat/1
  Delay1_bypass/1 -> in14_repeat/1
  From/1 -> slot_counter/1
  Goto/1 -> From/1
  Goto2/1 -> From25/1
  crp_out_delay/1 -> Delay1_lowered/1
  crp_out_delay1/1 -> Delay1_bypass/1
  in0_repeat/1 -> Delay_Switch/2, bypass_out/2
  in1_repeat/1 -> Delay_Switch/3, bypass_out/1
  in2_repeat/1 -> global_xor/1
  in3_repeat/1 -> global_xor/2
  in4_repeat/1 -> global_xor1/1
  in5_repeat/1 -> global_xor1/2
  in6_repeat/1 -> global_xor2/1
  in7_repeat/1 -> global_xor2/2
  in8_repeat/1 -> global_xor3/1
  in9_repeat/1 -> global_xor3/2
  in10_repeat/1 -> global_xor4/1
  in11_repeat/1 -> global_xor4/2
  in12_repeat/1 -> global_xor5/1
  in13_repeat/1 -> global_xor5/2
  in14_repeat/1 -> bypass_out/3
  delayMatch/1 -> out/1
  global_xor/1 -> global_xor9/1
  global_xor1/1 -> global_xor9/2
  global_xor9/1 -> global_xor11/1
  global_xor2/1 -> global_xor7/1
  global_xor3/1 -> global_xor7/2
  global_xor7/1 -> global_xor10/1
  global_xor4/1 -> global_xor8/1
  global_xor5/1 -> global_xor8/2
  global_xor8/1 -> global_xor10/2
  global_xor10/1 -> global_xor11/2
  global_xor11/1 -> Logical Operator/1
  Logical Operator/1 -> Delay_Switch/1
  Delay_Switch/1 -> crp_out_delay/1
  bypass_out/1 -> delayMatch/1, crp_out_delay1/1, Logical Operator/2
